simulink model "HW_02_DC_Machine_Sim"  (R2022b)
settings: Solver=VariableStepAuto  StartTime=0.0  StopTime=10.0  RelTol=1e-3
values from neighbouring files (symbols this model uses):
  pm_bp = 1e-4    (= 0.0001)    [HW1_2_Code_Hyeongmeen_Baik.m]
  pm_Jp = 1.34*1.355    (= 1.8157)    [HW1_2_Code_Hyeongmeen_Baik.m]
  pm_Ke = Kp_run02    (= 2.175)    [HW1_2_Code_Hyeongmeen_Baik.m]
  pm_Kt = Kp_run02    (= 2.175)    [HW1_2_Code_Hyeongmeen_Baik.m]
  pm_Lp = 0.013    [HW1_2_Code_Hyeongmeen_Baik.m]
  pm_Rp = 1.2*0.168    (= 0.2016)    [HW1_2_Code_Hyeongmeen_Baik.m]
  Ts_sim = 1e-6    (= 1e-06)    [HW1_2_Code_Hyeongmeen_Baik.m]
  Vstep = 5    [HW1_2_Code_Hyeongmeen_Baik.m]
settings Model: Creator=Hyeongmeen Baik  LastModifiedBy=Hyeongmeen Baik

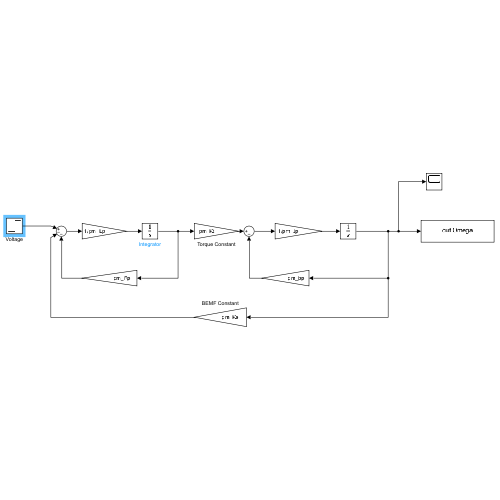
[thumbnail: Simulink's stored preview of the top-level diagram]
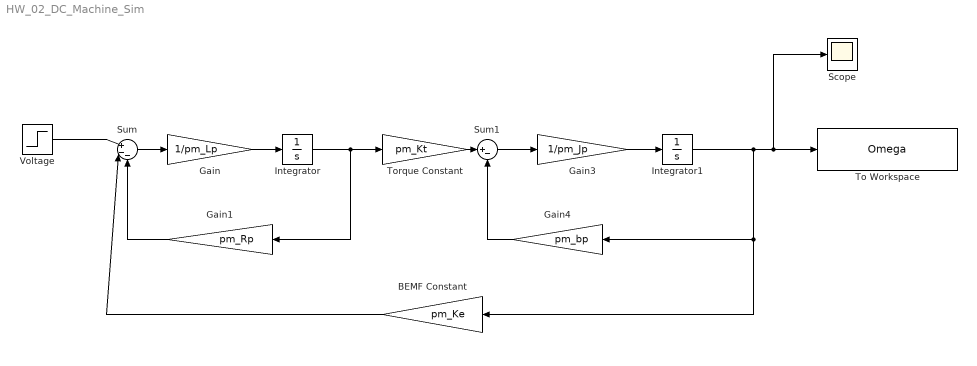
== system HW_02_DC_Machine_Sim ==
  BEMF Constant : Gain  Gain=pm_Ke
  Gain : Gain  Gain=1/pm_Lp
  Gain1 : Gain  Gain=pm_Rp
  Gain3 : Gain  Gain=1/pm_Jp
  Gain4 : Gain  Gain=pm_bp
  Integrator : Integrator
  Integrator1 : Integrator
  Scope : Scope
  Sum : Sum  Inputs=|+--
  Sum1 : Sum  Inputs=|+-
  To Workspace : ToWorkspace  VariableName=Omega  SaveFormat=Timeseries  SampleTime=Ts_sim
      settings: Save2DSignal=2-D array (concatenate along first dimension)
  Torque Constant : Gain  Gain=pm_Kt
  Voltage : Step  Time=0  After=Vstep  SampleTime=Ts_sim
  wires:
  Gain/1 -> Integrator/1
  Integrator/1 -> Gain1/1, Torque Constant/1
  Sum/1 -> Gain/1
  Gain1/1 -> Sum/3
  Torque Constant/1 -> Sum1/1
  Gain4/1 -> Sum1/2
  Sum1/1 -> Gain3/1
  Gain3/1 -> Integrator1/1
  Integrator1/1 -> Scope/1, To Workspace/1, BEMF Constant/1, Gain4/1
  BEMF Constant/1 -> Sum/2
  Voltage/1 -> Sum/1
